simulink model "automodel_Harness1"  (R2017b)
settings: Solver=VariableStepAuto  StartTime=0.0  StopTime=200  RelTol=1e-3
undefined symbols (not defined in the file): m, n, sigbuilder_block
settings Model: Creator=Kris  LastModifiedBy=Kris

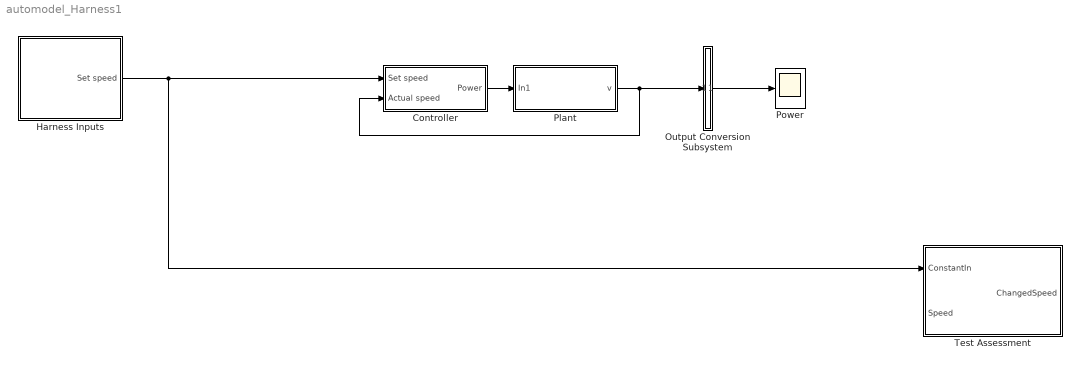
== system automodel_Harness1 ==
  Controller : Subsystem  Tag=__SL_testing_harness_stub_
  Harness Inputs : Subsystem  Tag=STV Subsys  LoadFcn=sigbuilder_block('load');  StartFcn=sigbuilder_block('start');  StopFcn=sigbuilder_block('stop');  ClipboardFcn=sigbuilder_block('clipboard');  mask(Sigbuilder block){tuvar=[0:10]}
      mask init:
      | if ~strcmp(get_param(bdroot(gcb),'SimulationStatus'),'stopped'),tuvar = sigbuilder_block('maskInit'); end
      settings: CopyFcn=sigbuilder_block('copy');  DeleteFcn=sigbuilder_block('delete');  ModelCloseFcn=sigbuilder_block('modelClose');  PreSaveFcn=sigbuilder_block('preSave');  PauseFcn=sigbuilder_block('pause');  ContinueFcn=sigbuilder_block('continue');  NameChangeFcn=sigbuilder_block('namechange');  OpenFcn=sigbuilder_block('open',[479.25 43.5 519.75 399.75 ]);  CloseFcn=sigbuilder_block('close');
      mask Display: plot(0, 0, 100, 100,[2, 2, 32, 32, 2], [68, 8, 8, 68, 68],[32, 2], [38, 38], [32, 19, 2],[53, 60, 44], [32, 17, 17, 2],[16, 16, 31, 31]);txt = getActiveGroup(gcbh);text(2, 100, txt,'verticalAlignment', 'top');
  Output Conversion Subsystem : Subsystem  Tag=__SLT_OCS__  Description=|
      | Signal spec.
      | and routing
      settings: AttributesFormatString=%<Description>
  Plant : Subsystem
  Power : Scope
  Test Assessment : Test Sequence  TreatAsAtomicUnit=on
  wires:
  Output Conversion Subsystem/1(Outport_1) -> Power/1
  Plant/1(v) -> Controller/2(Actual speed), Output Conversion Subsystem/1(Inport_1)
  Harness Inputs/1(Set speed) -> Controller/1(Set speed), Test Assessment/1(ConstantIn)
  Controller/1(Power) -> Plant/1(In1)

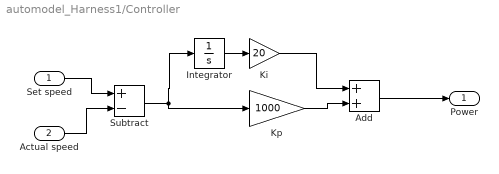
== system automodel_Harness1/Controller ==
  Set speed : Inport
  Actual speed : Inport  Port=2
  Add : Sum
  Integrator : Integrator
  Ki : Gain  Gain=20
  Kp : Gain  Gain=1000
  Subtract : Sum  Inputs=+-
  Power : Outport
  wires:
  Integrator/1 -> Ki/1
  Kp/1 -> Add/2
  Ki/1 -> Add/1
  Set speed/1 -> Subtract/1
  Subtract/1 -> Kp/1, Integrator/1
  Actual speed/1 -> Subtract/2
  Add/1 -> Power/1

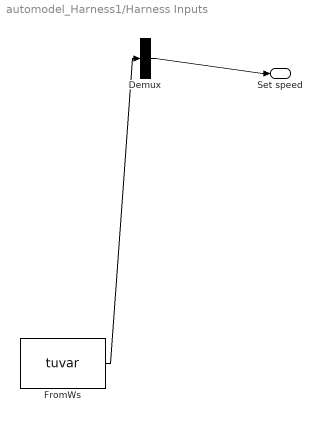
== system automodel_Harness1/Harness Inputs ==
  Demux : Demux  Tag=STV Demux  Outputs=1
  FromWs : FromWorkspace  Tag=STV FromWs  VariableName=tuvar  SampleTime=0
      SigBuilderData=|
      | dataSet.timeRange = [0 60]
      | dataSet.name = 'Group 1'
      | sbobj.Name = 'Signal Builder'
      | sbobj.Groups.Name = 'Group 1'
      | sbobj.Groups.Signals.Name = 'Set speed'
      | sbobj.Groups.Signals.XData = [0 24 24 36 36 60]
      | sbobj.Groups.Signals.YData = [40 40 50 50 40 40]
      | sbobj.Groups.TimeRange = [0 60]
  Set speed : Outport  Tag=STV Outport
  wires:
  FromWs/1 -> Demux/1
  Demux/1 -> Set speed/1

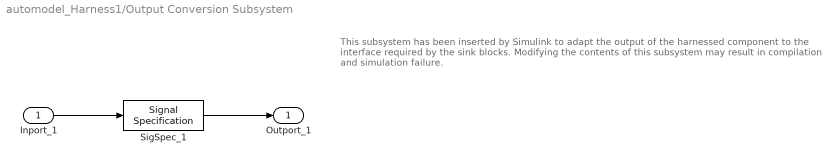
== system automodel_Harness1/Output Conversion Subsystem ==
  note: This subsystem has been inserted by Simulink to adapt the output of the harnessed component to the interface required by the sink blocks.
      |  Modifying the contents of this subsystem may result in compilation and simulation failure.
  Inport_1 : Inport
  SigSpec_1 : SignalSpecification  OutDataTypeStr=double  Dimensions=[1]
  Outport_1 : Outport
  wires:
  Inport_1/1 -> SigSpec_1/1
  SigSpec_1/1 -> Outport_1/1

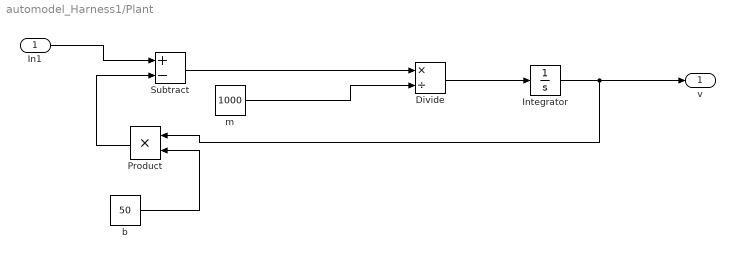
== system automodel_Harness1/Plant ==
  In1 : Inport
  Divide : Product  Inputs=*/
  Integrator : Integrator
  Product : Product
  Subtract : Sum  Inputs=+-
  b : Constant  Value=50
  m : Constant  Value=1000
  v : Outport
  wires:
  Product/1 -> Subtract/2
  b/1 -> Product/2
  Subtract/1 -> Divide/1
  m/1 -> Divide/2
  Integrator/1 -> Product/1, v/1
  In1/1 -> Subtract/1
  Divide/1 -> Integrator/1

== stateflow chart automodel_Harness1/Test Assessment ==
  settings: stateMachineType=SIMPLIFIED_MACHINE
  state ConstantCheck
    hasChanged(ConstantIn)
  state CheckSpeedLimit
    verify(Speed <=180)
    verify(Speed >= 40)
  state SettingTime
    ChangedSpeed = 0;
    state SettingTime_checkChange
      hasChanged(Speed)
    state SettingTime_wait
    state SettingTime_check
      verify(ConstantIn >= (Speed - 0.5))
      verify(ConstantIn <= (Speed + 0.5))
    (default) -> SettingTime_checkChange
    SettingTime_checkChange -> SettingTime_wait : [true
        | ]
    SettingTime_wait -> SettingTime_checkChange : [after(10,sec)
        | ]
  (default) -> ConstantCheck
  ConstantCheck -> CheckSpeedLimit : [false
      | ]
  CheckSpeedLimit -> ConstantCheck : [true
      | ]
  data: ConstantIn input; Speed input; ChangedSpeed output
